simulink library "Pressure_Drop_Ceta"  (R2018b)
settings: Solver=ode45  StartTime=0.0  StopTime=10.0  RelTol=1e-3  EnableMultiTasking=on
libraries: carnot x2
settings Model: Creator=drhf  LastModifiedBy=drhf
settings DataIOCC: LimitDataPoints=on  SaveFormat=Array  SignalLoggingSaveFormat=ModelDataLogs
settings OptimizationCC: ExpressionDepthLimit=2147483647  LifeSpan=inf
settings DebuggingCC: UnderspecifiedInitializationDetection=Classic  MergeDetectMultiDrivingBlocksExec=none  SolverPrmCheckMsg=warning  FcnCallInpInsideContextMsg=warning  StateNameClashWarn=warning  SFUnexpectedBacktrackingDiag=warning  SFNoUnconditionalDefaultTransitionDiag=warning  SFExecutionAtInitializationDiag=none
settings HardwareCC: ProdBitPerPointer=32  ProdBitPerSizeT=32  ProdBitPerPtrDiffT=32  ProdLargestAtomicFloat=None  ProdIntDivRoundTo=Undefined  ProdEndianess=Unspecified  ProdWordSize=32  ProdHWDeviceType=32-bit Generic
settings ModelReferenceCC: PropagateSignalLabelsOutOfModel=off
settings SFSimCC: SimUseLocalCustomCode=off
settings RTWCC: RTWUseLocalCustomCode=off
settings CodeAppCC: StateflowObjectComments=on
settings GRTTargetCC: TargetLangStandard=C89/C90 (ANSI)  GeneratePreprocessorConditionals=Disable all  CombineOutputUpdateFcns=off  GRTInterface=on
settings ConfigComp: CovMetricSettings=dw  CovHtmlReporting=on  CovSaveCumulativeToWorkspaceVar=on  CovSaveSingleToWorkspaceVar=on  CovExternalEMLEnable=off

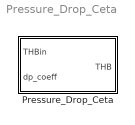
== system Pressure_Drop_Ceta ==
  Pressure_Drop_Ceta : Subsystem  mask(fixed pressure drop){con=101, lin=202, qua=303}
      mask prompts: con "c : constant (static) pressure drop in Pa"; lin "l : linear pressure drop Pa/(kg/s)"; qua "q : quadratic pressure drop Pa/(kg/s)²"
      mask help:
      | Calculates the pressure drop from a pressure drop coefficient ceta:
      | dp = ceta * density/2 * velocity²
      | Calculation is done for ID > 10000 (dp = f(l, q), c is neglected) and ID > 20000 (dp = f(c,l,q)).
      | Applied directly to the THB bus.
      mask Help: web(fullfile(path_carnot('help'),'Pressure_Drop_Ceta.html'),'-helpbrowser')

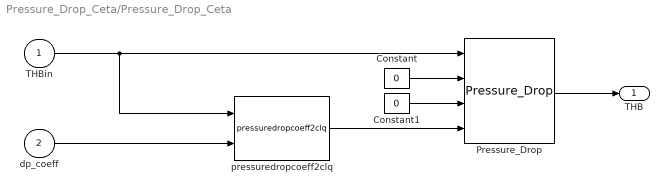
== system Pressure_Drop_Ceta/Pressure_Drop_Ceta ==
  THBin : Inport
  dp_coeff : Inport  Port=2
  Constant : Constant  Value=0
  Constant1 : Constant  Value=0
  Pressure_Drop : carnot/Basic/Pressure_Drop/Pressure_Drop
      settings: SourceProductName=Carnot
  pressuredropcoeff2clq : carnot/Basic/Pressure_Drop/pressuredropcoeff2clq
      settings: SourceProductName=Carnot
  THB : Outport
  wires:
  dp_coeff/1 -> pressuredropcoeff2clq/2
  pressuredropcoeff2clq/1 -> Pressure_Drop/4
  Constant1/1 -> Pressure_Drop/3
  Constant/1 -> Pressure_Drop/2
  THBin/1 -> Pressure_Drop/1, pressuredropcoeff2clq/1
  Pressure_Drop/1 -> THB/1
